simulink model "sampleModel1696"  (R2023a)
settings: Solver=VariableStepAuto  StartTime=0.0  StopTime=10.0  RelTol=1e-3
libraries: hdlsllib x3, simulink x2
settings Model: Creator=user1  LastModifiedBy=user1

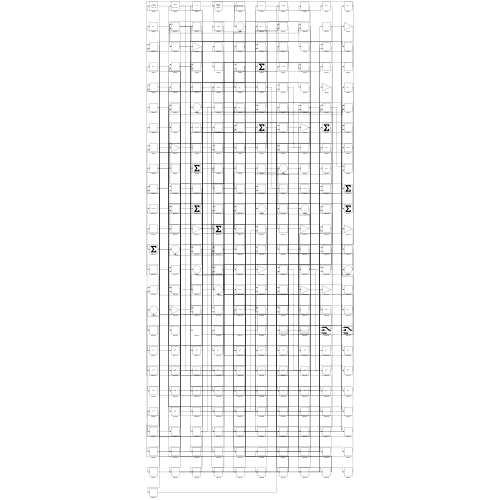
[thumbnail: Simulink's stored preview of the top-level diagram]
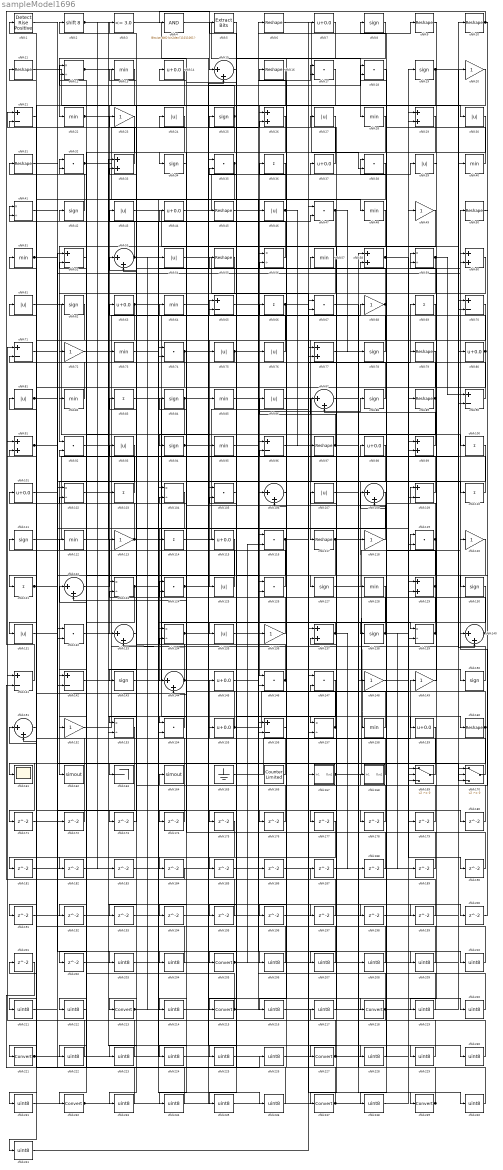
== system sampleModel1696 ==
  cfblk1 : hdlsllib/Logic and Bit Operations/Detect Rise Positive  vinit=0  OutDataTypeStr=boolean
  cfblk{6,9..11,16,31,45,50,55,79,89,97,117,160} (14 alike) : Reshape
  cfblk{36,66,69,83,100,103,110,114,121} (9 alike) : Sum  Inputs=+
  cfblk{7,14,37,44,63,80,98,101,115,145,155,159} (12 alike) : Bias  Bias=0.0  SaturateOnIntegerOverflow=off
  cfblk{12,41,56,59,102,104,123,134,139,153,157} (11 alike) : Product  Inputs=*/  RndMeth=Zero  SaturateOnIntegerOverflow=on
  cfblk{17..18,32,35,38,47,67,74,92,105,116,119,124,126,132,146..147,154} (18 alike) : DotProduct  OutDataTypeStr=Inherit: Inherit via internal rule
  cfblk{15,53,87,106,108,122,133,140,144,151} (10 alike) : Sum  Inputs=|++
  cfblk{24,27,30,39,43,46,54,61,75..76,81,86,93,107,125,131,135} (17 alike) : Abs  SaturateOnIntegerOverflow=off
  cfblk{21,52,65,70..71,90,96,109,141..142,156} (11 alike) : Sum  Inputs=+-
  cfblk{8,19,25,34,42,62,78,84,88,94,111,127,130,138,143,150} (16 alike) : Signum
  cfblk{13,22,28,40,48,51,57,64,73,82,85,95,112,128,158} (15 alike) : MinMax
  cfblk{20,23,49,68,72,113,118,120,136,148..149,152} (12 alike) : Gain
  cfblk{26,29,33,58,60,77,91,99,129,137} (10 alike) : Sum
  cfblk161 : Scope
  cfblk162 : ToWorkspace  VariableName=simout  SaveFormat=Timeseries  SampleTime=-1
  cfblk163 : Terminator
  cfblk164 : ToWorkspace  VariableName=simout  SaveFormat=Timeseries  SampleTime=-1
  cfblk165 : Ground
  cfblk166 : hdlsllib/Sources/Counter Limited  uplimit=7  tsamp=-1
  cfblk167 : Subsystem
      settings: LibrarySourceBlock=|
      | hdlsllib/Ports &
      | Subsystems/Subsystem
  cfblk168 : Subsystem
      settings: LibrarySourceBlock=|
      | hdlsllib/Ports &
      | Subsystems/Subsystem
  cfblk169 : Switch  SaturateOnIntegerOverflow=off  InputSameDT=off
  cfblk170 : Switch  SaturateOnIntegerOverflow=off  InputSameDT=off
  cfblk{171..202} (32 alike) : Delay  SampleTime=1
  cfblk2 : ArithShift  BitShiftNumber=8
  cfblk{203..204,206..212,214,216..217,219..220,222..226,228..231,233..236,238,240..241} (30 alike) : DataTypeConversion  OutDataTypeStr=uint8  SaturateOnIntegerOverflow=off  RndMeth=Floor
  cfblk{205,213,215,218,221,227,232,237,239} (9 alike) : DataTypeConversion  SaturateOnIntegerOverflow=off  RndMeth=Floor
  cfblk3 : hdlsllib/Logic and Bit Operations/Compare To Constant  relop=<=  const=3.0  OutDataTypeStr=boolean
  cfblk4 : simulink/Logic and Bit Operations/Bitwise Operator  logicop=AND  UseBitMask=on  BitMask=bin2dec('11011001')  BitMaskRealWorld=Stored Integer
      settings: LibrarySourceBlock=|
      | hdlsllib/Logic and Bit
      | Operations/Bitwise
      | Operator
  cfblk5 : simulink/Logic and Bit Operations/Extract Bits  bitsToExtract=Upper half  numBits=8  bitIdxRange=[0 7]  outScalingMode=Preserve fixed-point scaling
      settings: LibrarySourceBlock=|
      | hdlsllib/Logic and Bit
      | Operations/Extract Bits
  wires:
  cfblk19/1 -> cfblk146/1, cfblk140/2
  cfblk47/1 -> cfblk92/1, cfblk78/1
  cfblk9/1 -> cfblk127/1
  cfblk150/1 -> cfblk50/1
  cfblk166/1 -> cfblk81/1
  cfblk152/1 -> cfblk65/1
  cfblk10/1 -> cfblk164/1, cfblk4/1
  cfblk90/1 -> cfblk69/1
  cfblk37/1 -> cfblk25/1
  cfblk16/1 -> cfblk133/1
  cfblk167/1(Out1) -> cfblk119/1, cfblk207/1
  cfblk141/1 -> cfblk15/1
  cfblk122/1 -> cfblk113/1
  cfblk168/1(Out1) -> cfblk32/1
  cfblk103/1 -> cfblk93/1
  cfblk157/1 -> cfblk63/1, cfblk101/1
  cfblk69/1 -> cfblk117/1
  cfblk80/1 -> cfblk43/1, cfblk212/1
  cfblk134/1 -> cfblk156/2, cfblk214/1
  cfblk142/1 -> cfblk10/1
  cfblk143/1 -> cfblk68/1
  cfblk158/1 -> cfblk57/1
  cfblk109/1 -> cfblk38/1
  cfblk54/1 -> cfblk167/1(In1)
  cfblk76/1 -> cfblk23/1
  cfblk93/1 -> cfblk162/1
  cfblk117/1 -> cfblk158/1, cfblk196/1
  cfblk119/1 -> cfblk55/1, cfblk177/1
  cfblk30/1 -> cfblk76/1
  cfblk94/1 -> cfblk59/1, cfblk228/1
  cfblk61/1 -> cfblk103/1
  cfblk48/1 -> cfblk136/1
  cfblk68/1 -> cfblk82/1, cfblk115/1, cfblk2/1
  cfblk20/1 -> cfblk213/1
  cfblk111/1 -> cfblk40/1
  cfblk140/1 -> cfblk107/1, cfblk59/2
  cfblk51/1 -> cfblk131/1, cfblk109/2
  cfblk7/1 -> cfblk22/1
  cfblk110/1 -> cfblk92/2
  cfblk155/1 -> cfblk64/1, cfblk19/1
  cfblk65/1 -> cfblk146/2
  cfblk12/1 -> cfblk30/1, cfblk150/1, cfblk198/1
  cfblk36/1 -> cfblk142/1
  cfblk59/1 -> cfblk90/1, cfblk216/1
  cfblk156/1 -> cfblk16/1
  cfblk165/1 -> cfblk149/1
  cfblk6/1 -> cfblk38/2
  cfblk46/1 -> cfblk106/1, cfblk97/1
  cfblk106/1 -> cfblk36/1
  cfblk86/1 -> cfblk118/1
  cfblk87/1 -> cfblk148/1
  cfblk83/1 -> cfblk159/1
  cfblk55/1 -> cfblk62/1
  cfblk22/1 -> cfblk48/1, cfblk154/2
  cfblk18/1 -> cfblk138/1
  cfblk28/1 -> cfblk34/1
  cfblk127/1 -> cfblk120/1
  cfblk154/1 -> cfblk111/1
  cfblk113/1 -> cfblk139/1, cfblk12/1, cfblk47/2
  cfblk35/1 -> cfblk161/1, cfblk173/1
  cfblk98/1 -> cfblk227/1
  cfblk70/1 -> cfblk125/1
  cfblk170/1 -> cfblk145/1
  cfblk148/1 -> cfblk89/1
  cfblk147/1 -> cfblk215/1
  cfblk14/1 -> cfblk153/1
  cfblk151/1 -> cfblk221/1
  cfblk120/1 -> cfblk135/1
  cfblk11/1 -> cfblk75/1
  cfblk49/1 -> cfblk237/1
  cfblk32/1 -> cfblk6/1, cfblk156/1
  cfblk23/1 -> cfblk153/2
  cfblk74/1 -> cfblk121/1, cfblk178/1
  cfblk79/1 -> cfblk143/1
  cfblk126/1 -> cfblk53/1
  cfblk88/1 -> cfblk14/1
  cfblk25/1 -> cfblk12/2, cfblk193/1
  cfblk130/1 -> cfblk157/1
  cfblk96/1 -> cfblk218/1
  cfblk136/1 -> cfblk53/2
  cfblk78/1 -> cfblk66/1
  cfblk116/1 -> cfblk79/1, cfblk185/1
  cfblk53/1 -> cfblk41/1, cfblk170/2
  cfblk104/1 -> cfblk144/1
  cfblk52/1 -> cfblk232/1
  cfblk77/1 -> cfblk239/1
  cfblk133/1 -> cfblk3/1
  cfblk3/1 -> cfblk85/1
  cfblk97/1 -> cfblk100/1, cfblk86/1
  cfblk118/1 -> cfblk84/1
  cfblk8/1 -> cfblk106/2
  cfblk66/1 -> cfblk152/1, cfblk199/1
  cfblk135/1 -> cfblk88/1
  cfblk137/1 -> cfblk134/1, cfblk188/1
  cfblk139/1 -> cfblk124/1, cfblk27/1
  cfblk81/1 -> cfblk119/2, cfblk116/1, cfblk51/1
  cfblk149/1 -> cfblk109/1
  cfblk4/1 -> cfblk28/1
  cfblk27/1 -> cfblk114/1
  cfblk50/1 -> cfblk130/1
  cfblk89/1 -> cfblk61/1, cfblk222/1
  cfblk100/1 -> cfblk154/1
  cfblk138/1 -> cfblk24/1, cfblk189/1, cfblk190/1
  cfblk82/1 -> cfblk11/1
  cfblk114/1 -> cfblk7/1
  cfblk2/1 -> cfblk26/1, cfblk183/1
  cfblk43/1 -> cfblk70/2
  cfblk40/1 -> cfblk8/1
  cfblk56/1 -> cfblk41/2
  cfblk99/1 -> cfblk87/2
  cfblk58/1 -> cfblk170/3, cfblk238/1
  cfblk84/1 -> cfblk163/1, cfblk202/1, cfblk220/1
  cfblk63/1 -> cfblk142/2, cfblk60/1
  cfblk75/1 -> cfblk71/2, cfblk9/1
  cfblk45/1 -> cfblk17/1
  cfblk38/1 -> cfblk74/2
  cfblk129/1 -> cfblk108/2, cfblk174/1, cfblk175/1
  cfblk95/1 -> cfblk17/2
  cfblk123/1 -> cfblk192/1, cfblk236/1
  cfblk91/1 -> cfblk132/2, cfblk60/2
  cfblk101/1 -> cfblk110/1
  cfblk33/1 -> cfblk21/2
  cfblk73/1 -> cfblk95/1
  cfblk24/1 -> cfblk72/1
  cfblk108/1 -> cfblk123/1
  cfblk125/1 -> cfblk91/2
  cfblk64/1 -> cfblk160/1
  cfblk144/1 -> cfblk18/1, cfblk13/1, cfblk133/2
  cfblk105/1 -> cfblk205/1
  cfblk60/1 -> cfblk73/1
  cfblk42/1 -> cfblk31/1
  cfblk160/1 -> cfblk122/2, cfblk134/2, cfblk223/1
  cfblk121/1 -> cfblk126/1, cfblk206/1
  cfblk34/1 -> cfblk94/1
  cfblk169/1 -> cfblk112/1
  cfblk131/1 -> cfblk169/3
  cfblk146/1 -> cfblk83/1, cfblk56/2
  cfblk72/1 -> cfblk44/1
  cfblk44/1 -> cfblk39/1
  cfblk112/1 -> cfblk33/1
  cfblk17/1 -> cfblk56/1
  cfblk124/1 -> cfblk37/1, cfblk234/1
  cfblk159/1 -> cfblk171/1
  cfblk41/1 -> cfblk172/1
  cfblk172/1 -> cfblk21/1
  cfblk173/1 -> cfblk33/2
  cfblk174/1 -> cfblk91/1
  cfblk31/1 -> cfblk176/1
  cfblk176/1 -> cfblk123/2
  cfblk178/1 -> cfblk87/1
  cfblk179/1 -> cfblk18/2
  cfblk71/1 -> cfblk180/1
  cfblk180/1 -> cfblk70/1
  cfblk153/1 -> cfblk181/1
  cfblk181/1 -> cfblk74/1
  cfblk115/1 -> cfblk182/1
  cfblk182/1 -> cfblk15/2
  cfblk183/1 -> cfblk169/2
  cfblk26/1 -> cfblk184/1
  cfblk184/1 -> cfblk141/2
  cfblk185/1 -> cfblk129/2
  cfblk145/1 -> cfblk186/1
  cfblk188/1 -> cfblk104/2
  cfblk189/1 -> cfblk108/1
  cfblk190/1 -> cfblk144/2
  cfblk13/1 -> cfblk191/1
  cfblk191/1 -> cfblk99/1
  cfblk192/1 -> cfblk124/2
  cfblk193/1 -> cfblk139/2
  cfblk128/1 -> cfblk194/1
  cfblk194/1 -> cfblk157/2
  cfblk57/1 -> cfblk195/1
  cfblk195/1 -> cfblk132/1
  cfblk196/1 -> cfblk90/2
  cfblk92/1 -> cfblk197/1
  cfblk197/1 -> cfblk122/1
  cfblk198/1 -> cfblk58/2
  cfblk199/1 -> cfblk47/1
  cfblk107/1 -> cfblk200/1
  cfblk200/1 -> cfblk140/1
  cfblk202/1 -> cfblk46/1
  cfblk1/1 -> cfblk203/1
  cfblk203/1 -> cfblk80/1
  cfblk171/1 -> cfblk204/1
  cfblk204/1 -> cfblk1/1
  cfblk205/1 -> cfblk179/1, cfblk116/2
  cfblk206/1 -> cfblk105/1
  cfblk207/1 -> cfblk105/2
  cfblk187/1 -> cfblk208/1
  cfblk208/1 -> cfblk32/2
  cfblk85/1 -> cfblk209/1
  cfblk209/1 -> cfblk187/1
  cfblk102/1 -> cfblk210/1
  cfblk210/1 -> cfblk168/1(In1)
  cfblk62/1 -> cfblk211/1
  cfblk211/1 -> cfblk102/1
  cfblk212/1 -> cfblk102/2
  cfblk213/1 -> cfblk170/1, cfblk54/1
  cfblk214/1 -> cfblk20/1
  cfblk215/1 -> cfblk126/2, cfblk137/1, cfblk42/1
  cfblk216/1 -> cfblk147/1
  cfblk217/1 -> cfblk147/2
  cfblk218/1 -> cfblk217/1, cfblk137/2
  cfblk39/1 -> cfblk219/1
  cfblk219/1 -> cfblk96/1
  cfblk220/1 -> cfblk96/2
  cfblk221/1 -> cfblk35/1, cfblk104/1
  cfblk222/1 -> cfblk151/1
  cfblk223/1 -> cfblk151/2
  cfblk29/1 -> cfblk224/1
  cfblk224/1 -> cfblk169/1
  cfblk15/1 -> cfblk225/1
  cfblk225/1 -> cfblk29/1
  cfblk201/1 -> cfblk226/1
  cfblk226/1 -> cfblk29/2
  cfblk227/1 -> cfblk128/1, cfblk71/1
  cfblk228/1 -> cfblk98/1
  cfblk67/1 -> cfblk229/1
  cfblk229/1 -> cfblk141/1
  cfblk132/1 -> cfblk230/1
  cfblk230/1 -> cfblk67/1
  cfblk175/1 -> cfblk231/1
  cfblk231/1 -> cfblk67/2
  cfblk232/1 -> cfblk45/1, cfblk129/1
  cfblk177/1 -> cfblk233/1
  cfblk233/1 -> cfblk52/1
  cfblk234/1 -> cfblk52/2
  cfblk5/1 -> cfblk235/1
  cfblk235/1 -> cfblk99/2
  cfblk236/1 -> cfblk5/1
  cfblk237/1 -> cfblk201/1, cfblk26/2, cfblk155/1
  cfblk238/1 -> cfblk49/1
  cfblk239/1 -> cfblk58/1, cfblk35/2, cfblk65/2
  cfblk186/1 -> cfblk240/1
  cfblk240/1 -> cfblk77/1
  cfblk21/1 -> cfblk241/1
  cfblk241/1 -> cfblk77/2

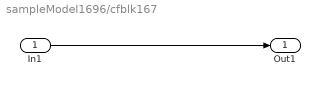
== system sampleModel1696/cfblk167 ==
  In1 : Inport
  Out1 : Outport
  wires:
  In1/1 -> Out1/1

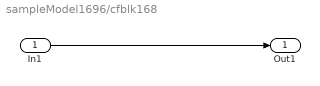
== system sampleModel1696/cfblk168 ==
  In1 : Inport
  Out1 : Outport
  wires:
  In1/1 -> Out1/1
